simulink model "New_Model_vmaRHTS_R2019b_2"  (R2023b)
settings: Solver=ode4  StartTime=0.0  StopTime=tend  FixedStep=dt  RelTol=1e-3
values from neighbouring files (symbols this model uses):
  Ag = zeros(15,1)    [New_Full.m]
  AgN = zeros(15,1)    [New_Ns1.m]    (also in New_Ns2.m)
  AgP = zeros(6,1)    [New_Ps.m]    (also in New_Ps1.m; New_Ps2.m)
  CNrt = CRrt    [New_Ns1.m]    (also in New_Ns2.m)
  CPrt = CRrt(locate2,locate2)    [New_Ps.m]    (also in New_Ps1.m = alphas(1) * MPrt + alphas(2) * KPrt; New_Ps2.m = alphas(1) * MPrt + alphas(2) * KPrt)
  CRrt = alphas(1) * MRrt + alphas(2) * KRrt    [New_Full.m]
  dt = 1/1024    (= 0.0009765625)    [New_Full.m]
  FN = zeros(15,1)    [New_Full.m]    (also in New_Ns1.m; New_Ns2.m)
  K_P1 = zeros(6,5)    [New_Guyan.m]
  K_P2 = zeros(6,1)    [New_Guyan.m]
  Kbar_inv = inv(Kbar)    [New_Full.m]
  KNbar_inv = inv(KNbar)    [New_Ns1.m]    (also in New_Ns2.m)
  KPbar_inv = inv(KPbar)    [New_Ps.m]    (also in New_Ps1.m; New_Ps2.m)
  KPrt = KRrt(locate2,locate2)    [New_Ps.m]    (also in New_Ps1.m = [2*Kc(4,4)+2*Kc(1,1)	Kc(4,6)+Kc(1,3)	Kc(4,6)+Kc(1,3); New_Ps2.m = [2*Kc(4,4)+2*Kc(1,1)	Kc(4,6)+Kc(1,3)	Kc(4,6)+Kc(1,3)	2*Kc(1,)
  KPuc = KPrt(locate5,locate4)    [New_Guyan.m]
  KPuu = KPrt(locate5,locate5)    [New_Guyan.m]
  KRrt = [4*Kc(4,4)+4*Kc(1,1)	Kc(4,6)+Kc(1,3)	Kc(4,6)+Kc(1,3)	Kc(4,6)+Kc(1,3)	Kc(4,6)+Kc(1,3)	4*Kc(1,4)	Kc(1,6)	Kc(1,6)	Kc(1,6)	Kc(1,6)	0	0	0	0	0 ... (first row only)    [New_Full.m]
  l = zeros(15,1)    [New_Full.m]
  lN = zeros(15,1)    [New_Ns1.m]    (also in New_Ns2.m)
  locate2 = [1,2,3]    [New_Ns1.m]    (also in New_Ns2.m = [1,2,3,6,7,8]; New_Ps.m = [1,2,3,6,7,8]; New_Ps1.m = [1,2,3,6,7,8]; New_Ps2.m = [1,2,3,6,7,8])
  locate3 = zeros(15,6)    [New_Ns1.m]    (also in New_Ns2.m)
  lP = zeros(6,1)    [New_Ps.m]    (also in New_Ps1.m; New_Ps2.m)
  MNrt = diag([M5 1e-5 M6 M3 M2 M1 M2 M3 M3 M2 M1 M2 M3 M3 M2])    [New_Ns1.m]    (also in New_Ns2.m = diag([M5 1e-5 M6 M3 M2 M5 1e-5 M6 M3 M2 M1 M2 M3 M3 M2]))
  MPrt = diag([M4 M2 M3 M4 M2 M3])    [New_Ps.m]    (also in New_Ps1.m = diag([M4 M2 M2]); New_Ps2.m = diag([M4 M2 M2 M4 M2 M2]))
  MPuu = MPrt(locate5,locate5)    [New_Guyan.m]
  MRrt = diag([M1 M2 M3 M3 M2 M1 M2 M3 M3 M2 M1 M2 M3 M3 M2])    [New_Full.m]
  Rbar = zeros(15,1)    [New_Full.m]
  RNbar = zeros(15,1)    [New_Ns1.m]    (also in New_Ns2.m)
  RPbar = zeros(6,1)    [New_Ps.m]    (also in New_Ps1.m; New_Ps2.m)
  tend = 40    [New_Full.m]
undefined symbols (not defined in the file or in its folder): a0, a1, a2, a3, a4, a5, a6, a7, Ag_tilde, C_tilde, Cp_tilde, CPren, Cren, EQ_intensity, EQ_sw, F_tilde, Klocate1, KN_tilde_inv, KNren_inv, Koo, Kot, Kp_tilde, KPren, Ksmn, Ksn, l_tilde, lren, M_tilde, Mp_tilde, MPren, Mren, Phi_u0, R_tilde, Rren, T
libraries: simulink x1, sldrtlib x1
(part 2 of 2)

== matlab function New_Model_vmaRHTS_R2019b_2/CBtest/ NUMERICAL SUBSTRUCTURE4/MATLAB Function1 ==
  data: U1 output; Vel1 output; Acc1 output; accel_grd input; KNbar_inv input; MNrt input; CNrt input; l input; RNbar input; Ag input; F input; F1 input; F2 input; T input; U0 input; Vel0 input; Acc0 input; a0 parameter; a1 parameter; a2 parameter; a3 parameter; a4 parameter; a5 parameter; a6 parameter; a7 parameter; RNbar output
function [U1,Vel1,Acc1,RNbar]=fcn2(accel_grd,KNbar_inv, MNrt, CNrt,l,RNbar,Ag,F,F1,F2,T,...
    U0,Vel0,Acc0, a0, a1, a2, a3, a4, a5, a6, a7)
             
    % 该求解方法为 Newmark-β法        
    % ============================
	% *  Update next iteration   *
	% ============================
    ndof = length(KNbar_inv);
    U1   = zeros(ndof,1);
    Vel1 = zeros(ndof,1);
    Acc1 = zeros(ndof,1);
    
    F1 = F;
    % ============================
	% *  Feedback Force / Moment *
	% ============================
%     F(27) = -FB_force;
%     F(14) = -FB_moment;

    % ==========================
	% *     Update Matrices    *
	% ==========================
    Ag  = accel_grd * l;
   	% ==========================
	% * 	  Form Rbar  	   *
	% ==========================
	%RNbar = ( (MNrt * ((a0*U0)+(a2*Vel0)+(a3*Acc0))) + ...
	%	     (CNrt * ((a1*U0)+(a4*Vel0)+(a5*Acc0))) -F1-  (MNrt * Ag) );

    RNbar = ( (MNrt * ((a0*U0)+(a2*Vel0)+(a3*Acc0))) + ...
		     (CNrt * ((a1*U0)+(a4*Vel0)+(a5*Acc0))) -F1-  (MNrt * Ag) );
    
    % ==========================
	% * Solve for Displacement *
	% ==========================
	U1 = KNbar_inv * RNbar;
    
	% ============================
	% * Compute Velocity & Accel *
	% ============================
	Acc1=a0*(U1-U0)-a2*Vel0-a3*Acc0;
	Vel1=Vel0+a7*Acc1+a6*Acc0;

end
